simulink model "subscribe_model"  (R2015b)
settings: Solver=ode5  StartTime=0.0  StopTime=inf  FixedStep=0.0005  RelTol=1e-3
libraries: robotlib x4, aerolibanimutils x1
settings Model: Creator=root  LastModifiedBy=root

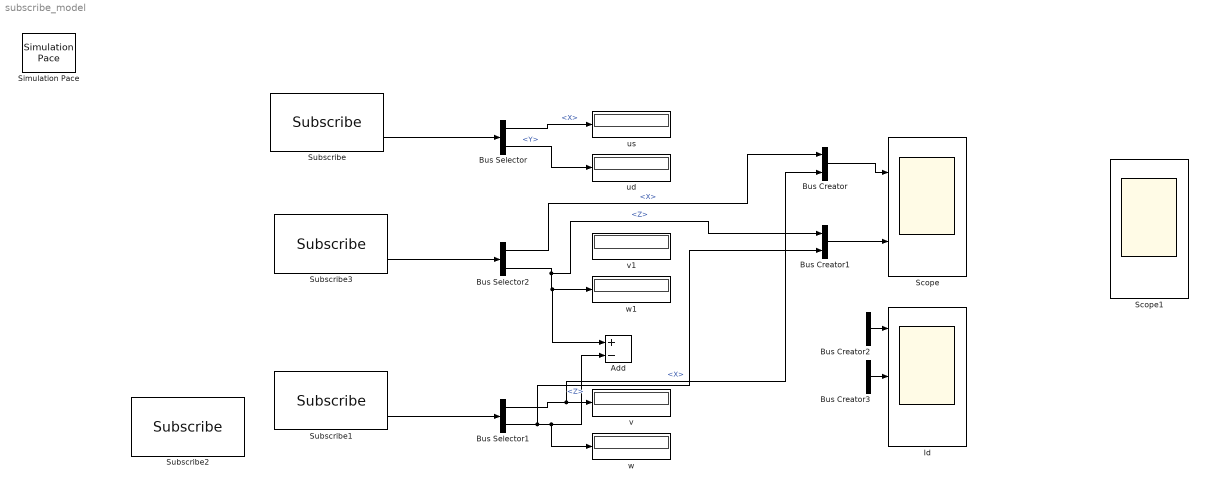
== system subscribe_model ==
  Add : Sum  Inputs=+-
  Bus Creator{,1..3} (4 alike) : BusCreator  Inputs=2
  Bus Selector : BusSelector  OutputSignals=X,Y
  Bus Selector1 : BusSelector  OutputSignals=Linear.X,Angular.Z
  Bus Selector2 : BusSelector  OutputSignals=Linear.X,Angular.Z
  Id : Scope  NumInputPorts=3
  Scope : Scope  NumInputPorts=2
  Scope1 : Scope  NumInputPorts=3
  Simulation Pace : aerolibanimutils/Simulation Pace  SimulationPace=1  SleepMode=MATLAB Thread  OutputPaceError=off  SampleTime=-1
  Subscribe : robotlib/Subscribe  SourceLibraryInfo=This block requires Robotics System Toolbox  topicSource=Select from ROS network  topic=/andbot/cmd_us_ud  messageType=geometry_msgs/Vector3  sampleTime=-1  messageQueueLength=1
  Subscribe1 : robotlib/Subscribe  SourceLibraryInfo=This block requires Robotics System Toolbox  topicSource=Select from ROS network  topic=/andbot/feedback_vel  messageType=geometry_msgs/Twist  sampleTime=-1  messageQueueLength=1
  Subscribe2 : robotlib/Subscribe  SourceLibraryInfo=This block requires Robotics System Toolbox  topicSource=Select from ROS network  topic=/andbot/feedback_vel  messageType=geometry_msgs/Twist  sampleTime=-1  messageQueueLength=1
  Subscribe3 : robotlib/Subscribe  SourceLibraryInfo=This block requires Robotics System Toolbox  topicSource=Select from ROS network  topic=/andbot/cmd_vel  messageType=geometry_msgs/Twist  sampleTime=-1  messageQueueLength=1
  ud : Display
  us : Display
  v : Display
  v1 : Display
  w : Display
  w1 : Display
  wires:
  Subscribe/2 -> Bus Selector/1
  Bus Selector/1 -> us/1  "<X>"
  Bus Selector/2 -> ud/1  "<Y>"
  Subscribe1/2 -> Bus Selector1/1
  Bus Selector1/1 -> Bus Creator/2, v/1  "<X>"
  Bus Selector1/2 -> Bus Creator1/2, Add/2, w/1  "<Z>"
  Bus Creator/1 -> Scope/1
  Subscribe3/2 -> Bus Selector2/1
  Bus Selector2/2 -> Bus Creator1/1, Add/1, w1/1  "<Z>"
  Bus Creator2/1 -> Id/1
  Bus Creator3/1 -> Id/2
  Bus Selector2/1 -> Bus Creator/1  "<X>"
  Bus Creator1/1 -> Scope/2
